simulink library "Damper_Basics"  (R2026a)
settings: Solver=VariableStepAuto
undefined symbols (not defined in the file): Damper, Vehicle
libraries: fl_lib x13, nesl_utility x8, $bdroot x6, sdl_lib x1
Description:
  | Component of Simscape Vehicle Templates Library
  | 
  | Copyright 2018-2026 The MathWorks, Inc.
settings Model: Creator=smiller  LastModifiedBy=smiller

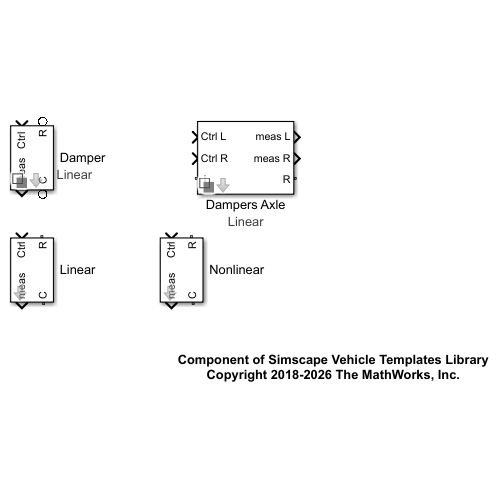
[thumbnail: Simulink's stored preview of the top-level diagram]
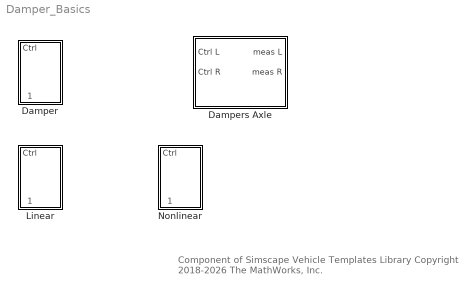
== system Damper_Basics ==
  note: Component of Simscape Vehicle Templates Library
      | Copyright 2018-2026 The MathWorks, Inc.
  Damper : Subsystem  Variant=on  VariantControlMode=label  VariantControl=Variant1  LabelModeActiveChoice=Linear  mask(Variants for Damper){Damper=Vehicle.Chassis.Damper.Axle1, VariantLabel=Vehicle.Chassis.Damper.Axle1.class.Value, InitTriggerDropdown=1}
      mask prompts: Damper "Damper Parameters"; VariantLabel "Variant Label"; InitTriggerDropdown "Initialization Trigger Dropdown"
      mask help: Select option and provide parameters for damper. Option is chosen by string provided in Variant Label. The parameters for the selected option is contained in Damper data structure.
      mask init:
      | curblk = gcb;
      | 
      | % Set variant for this block 
      | set_param(curblk,'LabelModeActiveChoice',VariantLabel);
      | 
      | % Trigger Mask Initialization for 
      | % variant subsystems below this level
      | sm_car_lib_maskInitTrigger(curblk);
      settings: AttributesFormatString=%<ActiveVariant>
      mask TypeOptions InitTriggerDropdown: 0 | 1
      mask Display: disp(' ')
  Dampers Axle : Subsystem  Variant=on  VariantControlMode=label  VariantControl=Variant1  LabelModeActiveChoice=Linear  mask(Variants for Dampers){Damper=Vehicle.Chassis.Damper.Axle1, VariantLabel=Vehicle.Chassis.Damper.Axle1.class.Value, InitTriggerDropdown=1}
      mask prompts: Damper "Damper Parameters"; VariantLabel "Variant Label"; InitTriggerDropdown "Initialization Trigger Dropdown"
      mask help: Select option and provide parameters for left and right dampers. Option is chosen by string provided in Variant Label. The parameters for the selected option is contained in Damper data structure.
      mask init:
      | curblk = gcb;
      | 
      | % Set variant for this block 
      | set_param(curblk,'LabelModeActiveChoice',VariantLabel);
      | 
      | % Trigger Mask Initialization for 
      | % variant subsystems below this level
      | sm_car_lib_maskInitTrigger(curblk);
      settings: AttributesFormatString=%<ActiveVariant>
      mask TypeOptions InitTriggerDropdown: 0 | 1
      mask Display: disp(' ')
  Linear : Subsystem  VariantControl=Linear  mask(Linear Damper with Bumpstop){dam_b=Damper.Damping.d.Value, hp_dpr_top=Damper.Damping.sTop.Value, hp_dpr_bot=Damper.Damping.sBottom.Value, bs_lim_upper=Damper.Endstop.xMax.Value, bs_lim_lower=Damper.Endstop.xMin.Value, bs_k_upper=Damper.Endstop.KxMax.Value, bs_k_lower=Damper.Endstop.KxMin.Value, bs_b_upper=Damper.Endstop.dxMax.Value, bs_b_lower=Damper.Endstop.dxMin.Value, bs_region=Damper.Endstop.xTransition.Value}
      mask prompts: dam_b "Damper (N/(m/s))"; hp_dpr_top "HP Damper Top [xyz] (m)"; hp_dpr_bot "HP Damper Bottom [xyz] (m)"; bs_region "Transition Region (m)"
      mask help: Linear damper with bumpstop at top and bottom.
      mask init:
      | dam_x0 = norm(hp_dpr_top - hp_dpr_bot);
      mask TypeOptions dam_b: Damper/D
      mask DialogControl text_bumpstop_upper Prompt: Upper
      mask DialogControl text_bumpstop_lower Prompt: Lower
      mask DialogControl text_bumpstop_limit Prompt: Limit (m)
      mask DialogControl text_bumpstop_k Prompt: Stiffness (N/m)
      mask DialogControl text_bumpstop_b Prompt: Damping  (N/(m/s))
  Nonlinear : Subsystem  VariantControl=Nonlinear  mask(Nonlinear Damper with Bumpstop){velocity_vector=Damper.Damping.vDamper.Value, force_vector=Damper.Damping.fDamper.Value, hp_dpr_top=Damper.Damping.sTop.Value, hp_dpr_bot=Damper.Damping.sBottom.Value, bs_lim_upper=Damper.Endstop.xMax.Value, bs_lim_lower=Damper.Endstop.xMin.Value, bs_k_upper=Damper.Endstop.KxMax.Value, bs_k_lower=Damper.Endstop.KxMin.Value, bs_b_upper=Damper.Endstop.dxMax.Value, bs_b_lower=Damper.Endstop.dxMin.Value, bs_region=Damper.Endstop.xTransition.Value}
      mask prompts: velocity_vector "Velocity vector"; force_vector "Force vector"; hp_dpr_top "HP Damper Top [xyz] (m)"; hp_dpr_bot "HP Damper Bottom [xyz] (m)"; bs_region "Transition Region (m)"
      mask help: Damper with damping coefficient specified as a lookup table in parallel with a bumpstop.
      mask init:
      | dam_x0 = norm(hp_dpr_top - hp_dpr_bot);
      mask TypeOptions velocity_vector: Damper/velocity_vector
      mask TypeOptions force_vector: Damper/force_vector
      mask DialogControl text_bumpstop_upper Prompt: Upper
      mask DialogControl text_bumpstop_lower Prompt: Lower
      mask DialogControl text_bumpstop_limit Prompt: Limit (m)
      mask DialogControl text_bumpstop_k Prompt: Stiffness (N/m)
      mask DialogControl text_bumpstop_b Prompt: Damping  (N/(m/s))

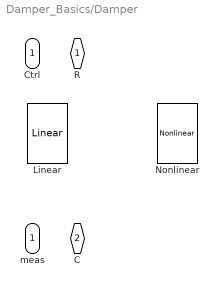
== system Damper_Basics/Damper ==
  "Ctrl " : Inport
  Linear : $bdroot/Linear  VariantControl=Linear  dam_b=Damper.Damping.d.Value  hp_dpr_top=Damper.Damping.sTop.Value  hp_dpr_bot=Damper.Damping.sBottom.Value  bs_lim_upper=Damper.Endstop.xMax.Value  bs_lim_lower=Damper.Endstop.xMin.Value  bs_k_upper=Damper.Endstop.KxMax.Value  bs_k_lower=Damper.Endstop.KxMin.Value  bs_b_upper=Damper.Endstop.dxMax.Value  bs_b_lower=Damper.Endstop.dxMin.Value  bs_region=Damper.Endstop.xTransition.Value
  Nonlinear : $bdroot/Nonlinear  VariantControl=Nonlinear  velocity_vector=Damper.Damping.vDamper.Value  force_vector=Damper.Damping.fDamper.Value  hp_dpr_top=Damper.Damping.sTop.Value  hp_dpr_bot=Damper.Damping.sBottom.Value  bs_lim_upper=Damper.Endstop.xMax.Value  bs_lim_lower=Damper.Endstop.xMin.Value  bs_k_upper=Damper.Endstop.KxMax.Value  bs_k_lower=Damper.Endstop.KxMin.Value  bs_b_upper=Damper.Endstop.dxMax.Value  bs_b_lower=Damper.Endstop.dxMin.Value  bs_region=Damper.Endstop.xTransition.Value
  " R" : PMIOPort  Side=Left
  " C" : PMIOPort  Port=2  Side=Right
  " meas" : Outport  VectorParamsAs1DForOutWhenUnconnected=off

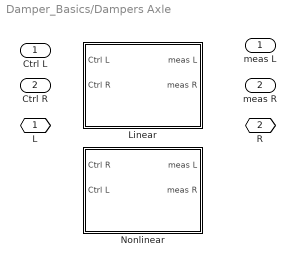
== system Damper_Basics/Dampers Axle ==
  "Ctrl L " : Inport
  "Ctrl R " : Inport  Port=2
  Linear : Subsystem  VariantControl=Linear
  Nonlinear : Subsystem  VariantControl=Nonlinear
  " L" : PMIOPort  Side=Left
  " R" : PMIOPort  Port=2  Side=Right
  " meas L" : Outport  VectorParamsAs1DForOutWhenUnconnected=off
  " meas R" : Outport  Port=2  VectorParamsAs1DForOutWhenUnconnected=off

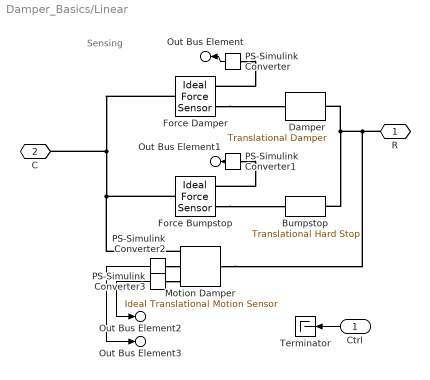
== system Damper_Basics/Linear ==
  note: Sensing
  Ctrl : Inport
  Bumpstop : fl_lib/Mechanical/Translational Elements/Translational Hard Stop  upper_bnd=bs_lim_upper m  lower_bnd=bs_lim_lower m  model=1  stiff_up=bs_k_upper N/m  stiff_low=bs_k_lower N/m  D_up=bs_b_upper N/(m/s)  D_low=bs_b_lower N/(m/s)  transition=bs_region m  coeff_rest=0.7  v_tol=0.001 m/s  f_tol=0.001 N  v_specify=off  v_priority=None  v=0 m/s  v_nominal_specify=off  v_nominal_value=1  v_nominal_unit=m/s  f_specify=off  f_priority=None  f=0 N  f_nominal_specify=off  f_nominal_value=1  f_nominal_unit=N  x_specify=off  x_priority=High  x=0 m  x_nominal_specify=off  x_nominal_value=1  x_nominal_unit=m  M_specify=off  M_priority=None  M=0
  Damper : fl_lib/Mechanical/Translational Elements/Translational Damper  D=dam_b N/(m/s)  v_specify=off  v_priority=None  v=0 m/s  v_nominal_specify=off  v_nominal_value=1  v_nominal_unit=m/s  f_specify=off  f_priority=None  f=0 N  f_nominal_specify=off  f_nominal_value=1  f_nominal_unit=N
  Force Bumpstop : fl_lib/Mechanical/Mechanical Sensors/Ideal Force Sensor
  Force Damper : fl_lib/Mechanical/Mechanical Sensors/Ideal Force Sensor
  Motion Damper : fl_lib/Mechanical/Mechanical Sensors/Ideal Translational Motion Sensor  reference=foundation.enum.MeasurementReference.difference  acceleration_port=false  velocity_port=true  position_port=true  offset=dam_x0 m
  PS-Simulink Converter : nesl_utility/PS-Simulink Converter  PhysicalDomain=network_engine_domain  SubClassName=ps_output  LeftPortType=input  RightPortType=output  PseudoPeriodic=off  Frequencies=[]  VectorFormat=1-D array  Unit=N  AffineConversion=off
  PS-Simulink Converter1 : nesl_utility/PS-Simulink Converter  PhysicalDomain=network_engine_domain  SubClassName=ps_output  LeftPortType=input  RightPortType=output  PseudoPeriodic=off  Frequencies=[]  VectorFormat=1-D array  Unit=N  AffineConversion=off
  PS-Simulink Converter2 : nesl_utility/PS-Simulink Converter  PhysicalDomain=network_engine_domain  SubClassName=ps_output  LeftPortType=input  RightPortType=output  PseudoPeriodic=off  Frequencies=[]  VectorFormat=1-D array  Unit=m/s  AffineConversion=off
  PS-Simulink Converter3 : nesl_utility/PS-Simulink Converter  PhysicalDomain=network_engine_domain  SubClassName=ps_output  LeftPortType=input  RightPortType=output  PseudoPeriodic=off  Frequencies=[]  VectorFormat=1-D array  Unit=m  AffineConversion=off
  Terminator : Terminator
  R : PMIOPort  Side=Left
  C : PMIOPort  Port=2  Side=Right
  Out Bus Element : Outport  VectorParamsAs1DForOutWhenUnconnected=off  PortName=meas  Element=FDamper
  Out Bus Element1 : Outport  VectorParamsAs1DForOutWhenUnconnected=off  PortName=meas  Element=FBumpstop
  Out Bus Element2 : Outport  VectorParamsAs1DForOutWhenUnconnected=off  PortName=meas  Element=xDamper
  Out Bus Element3 : Outport  VectorParamsAs1DForOutWhenUnconnected=off  PortName=meas  Element=vDamper
  wires:
  Ctrl/1 -> Terminator/1
  PS-Simulink Converter/1 -> Out Bus Element/1
  PS-Simulink Converter2/1 -> Out Bus Element3/1
  PS-Simulink Converter3/1 -> Out Bus Element2/1
  PS-Simulink Converter1/1 -> Out Bus Element1/1
  connections:
  Motion Damper/RConn1 -- Force Bumpstop/LConn1 -- C/RConn1 -- Force Damper/LConn1
  PS-Simulink Converter2/LConn1 -- Motion Damper/RConn2
  PS-Simulink Converter1/LConn1 -- Force Bumpstop/RConn2
  PS-Simulink Converter3/LConn1 -- Motion Damper/RConn3
  PS-Simulink Converter/LConn1 -- Force Damper/RConn2
  Force Bumpstop/RConn1 -- Bumpstop/RConn1
  Force Damper/RConn1 -- Damper/RConn1
  Damper/LConn1 -- Bumpstop/LConn1 -- Motion Damper/LConn1 -- R/RConn1

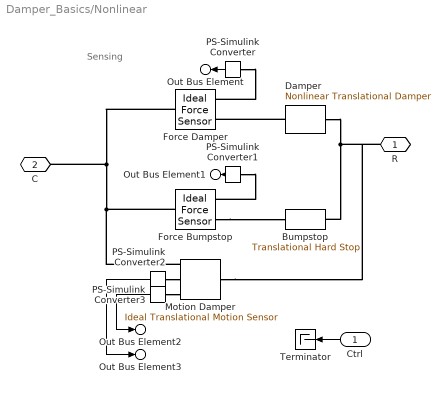
== system Damper_Basics/Nonlinear ==
  note: Sensing
  Ctrl : Inport
  Bumpstop : fl_lib/Mechanical/Translational Elements/Translational Hard Stop  upper_bnd=bs_lim_upper m  lower_bnd=bs_lim_lower m  model=1  stiff_up=bs_k_upper N/m  stiff_low=bs_k_lower N/m  D_up=bs_b_upper N/(m/s)  D_low=bs_b_lower N/(m/s)  transition=bs_region m  coeff_rest=0.7  v_tol=0.001 m/s  f_tol=0.001 N  v_specify=off  v_priority=None  v=0 m/s  v_nominal_specify=off  v_nominal_value=1  v_nominal_unit=m/s  f_specify=off  f_priority=None  f=0 N  f_nominal_specify=off  f_nominal_value=1  f_nominal_unit=N  x_specify=off  x_priority=High  x=0 m  x_nominal_specify=off  x_nominal_value=1  x_nominal_unit=m  M_specify=off  M_priority=None  M=0
  Damper : sdl_lib/Couplings & Drives/Springs & Dampers/Nonlinear Translational Damper  parameterization=2  symmetry=1  coefficient_vector=[10, 0, 1, 0, .1] N/(m/s)  extension_coefficient_vector=[10, 0, 1, 0, .1] N/(m/s)  contraction_coefficient_vector=[100, -1, 10, 0, 0] N/(m/s)  velocity_vector=velocity_vector m/s  force_vector=force_vector N  interp_method=simscape.enum.interpolation.linear  extrap_method=simscape.enum.extrapolation.linear
  Force Bumpstop : fl_lib/Mechanical/Mechanical Sensors/Ideal Force Sensor
  Force Damper : fl_lib/Mechanical/Mechanical Sensors/Ideal Force Sensor
  Motion Damper : fl_lib/Mechanical/Mechanical Sensors/Ideal Translational Motion Sensor  reference=foundation.enum.MeasurementReference.difference  acceleration_port=false  velocity_port=true  position_port=true  offset=dam_x0 m
  PS-Simulink Converter : nesl_utility/PS-Simulink Converter  PhysicalDomain=network_engine_domain  SubClassName=ps_output  LeftPortType=input  RightPortType=output  PseudoPeriodic=off  Frequencies=[]  VectorFormat=1-D array  Unit=N  AffineConversion=off
  PS-Simulink Converter1 : nesl_utility/PS-Simulink Converter  PhysicalDomain=network_engine_domain  SubClassName=ps_output  LeftPortType=input  RightPortType=output  PseudoPeriodic=off  Frequencies=[]  VectorFormat=1-D array  Unit=N  AffineConversion=off
  PS-Simulink Converter2 : nesl_utility/PS-Simulink Converter  PhysicalDomain=network_engine_domain  SubClassName=ps_output  LeftPortType=input  RightPortType=output  PseudoPeriodic=off  Frequencies=[]  VectorFormat=1-D array  Unit=m/s  AffineConversion=off
  PS-Simulink Converter3 : nesl_utility/PS-Simulink Converter  PhysicalDomain=network_engine_domain  SubClassName=ps_output  LeftPortType=input  RightPortType=output  PseudoPeriodic=off  Frequencies=[]  VectorFormat=1-D array  Unit=m  AffineConversion=off
  Terminator : Terminator
  R : PMIOPort  Side=Left
  C : PMIOPort  Port=2  Side=Right
  Out Bus Element : Outport  VectorParamsAs1DForOutWhenUnconnected=off  PortName=meas  Element=FDamper
  Out Bus Element1 : Outport  VectorParamsAs1DForOutWhenUnconnected=off  PortName=meas  Element=FBumpstop
  Out Bus Element2 : Outport  VectorParamsAs1DForOutWhenUnconnected=off  PortName=meas  Element=xDamper
  Out Bus Element3 : Outport  VectorParamsAs1DForOutWhenUnconnected=off  PortName=meas  Element=vDamper
  wires:
  PS-Simulink Converter1/1 -> Out Bus Element1/1
  PS-Simulink Converter3/1 -> Out Bus Element2/1
  PS-Simulink Converter2/1 -> Out Bus Element3/1
  PS-Simulink Converter/1 -> Out Bus Element/1
  Ctrl/1 -> Terminator/1
  connections:
  Damper/LConn1 -- R/RConn1 -- Motion Damper/LConn1 -- Bumpstop/LConn1
  Damper/RConn1 -- Force Damper/RConn1
  Force Bumpstop/RConn1 -- Bumpstop/RConn1
  PS-Simulink Converter/LConn1 -- Force Damper/RConn2
  PS-Simulink Converter3/LConn1 -- Motion Damper/RConn3
  PS-Simulink Converter1/LConn1 -- Force Bumpstop/RConn2
  PS-Simulink Converter2/LConn1 -- Motion Damper/RConn2
  Force Damper/LConn1 -- C/RConn1 -- Force Bumpstop/LConn1 -- Motion Damper/RConn1

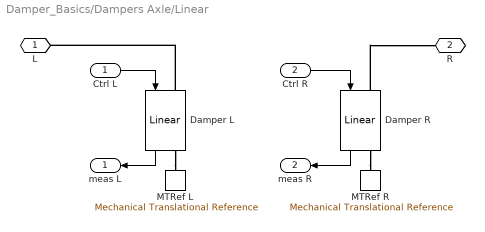
== system Damper_Basics/Dampers Axle/Linear ==
  Ctrl L : Inport
  Ctrl R : Inport  Port=2
  Damper L : $bdroot/Linear  VariantControl=Linear  dam_b=Damper.Damping.d.Value  hp_dpr_top=Damper.Damping.sTop.Value  hp_dpr_bot=Damper.Damping.sBottom.Value  bs_lim_upper=Damper.Endstop.xMax.Value  bs_lim_lower=Damper.Endstop.xMin.Value  bs_k_upper=Damper.Endstop.KxMax.Value  bs_k_lower=Damper.Endstop.KxMin.Value  bs_b_upper=Damper.Endstop.dxMax.Value  bs_b_lower=Damper.Endstop.dxMin.Value  bs_region=Damper.Endstop.xTransition.Value
  Damper R : $bdroot/Linear  VariantControl=Linear  dam_b=Damper.Damping.d.Value  hp_dpr_top=Damper.Damping.sTop.Value  hp_dpr_bot=Damper.Damping.sBottom.Value  bs_lim_upper=Damper.Endstop.xMax.Value  bs_lim_lower=Damper.Endstop.xMin.Value  bs_k_upper=Damper.Endstop.KxMax.Value  bs_k_lower=Damper.Endstop.KxMin.Value  bs_b_upper=Damper.Endstop.dxMax.Value  bs_b_lower=Damper.Endstop.dxMin.Value  bs_region=Damper.Endstop.xTransition.Value
  MTRef L : fl_lib/Mechanical/Translational Elements/Mechanical Translational Reference
  MTRef R : fl_lib/Mechanical/Translational Elements/Mechanical Translational Reference
  " L" : PMIOPort  Side=Left
  " R" : PMIOPort  Port=2  Side=Right
  meas L : Outport  VectorParamsAs1DForOutWhenUnconnected=off
  meas R : Outport  Port=2  VectorParamsAs1DForOutWhenUnconnected=off
  wires:
  Damper L/1 -> meas L/1
  Ctrl L/1 -> Damper L/1
  Ctrl R/1 -> Damper R/1
  Damper R/1 -> meas R/1
  connections:
  Damper L/RConn1 -- MTRef L/LConn1
  Damper R/LConn1 -- " R"/RConn1
  Damper R/RConn1 -- MTRef R/LConn1
  Damper L/LConn1 -- " L"/RConn1

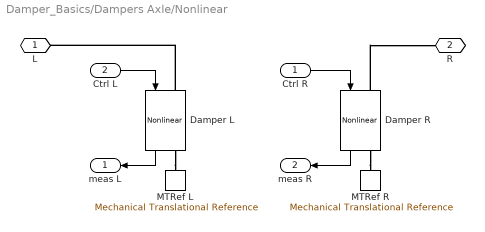
== system Damper_Basics/Dampers Axle/Nonlinear ==
  Ctrl R : Inport
  Ctrl L : Inport  Port=2
  Damper L : $bdroot/Nonlinear  VariantControl=Nonlinear  velocity_vector=Damper.Damping.vDamper.Value  force_vector=Damper.Damping.fDamper.Value  hp_dpr_top=Damper.Damping.sTop.Value  hp_dpr_bot=Damper.Damping.sBottom.Value  bs_lim_upper=Damper.Endstop.xMax.Value  bs_lim_lower=Damper.Endstop.xMin.Value  bs_k_upper=Damper.Endstop.KxMax.Value  bs_k_lower=Damper.Endstop.KxMin.Value  bs_b_upper=Damper.Endstop.dxMax.Value  bs_b_lower=Damper.Endstop.dxMin.Value  bs_region=Damper.Endstop.xTransition.Value
  Damper R : $bdroot/Nonlinear  VariantControl=Nonlinear  velocity_vector=Damper.Damping.vDamper.Value  force_vector=Damper.Damping.fDamper.Value  hp_dpr_top=Damper.Damping.sTop.Value  hp_dpr_bot=Damper.Damping.sBottom.Value  bs_lim_upper=Damper.Endstop.xMax.Value  bs_lim_lower=Damper.Endstop.xMin.Value  bs_k_upper=Damper.Endstop.KxMax.Value  bs_k_lower=Damper.Endstop.KxMin.Value  bs_b_upper=Damper.Endstop.dxMax.Value  bs_b_lower=Damper.Endstop.dxMin.Value  bs_region=Damper.Endstop.xTransition.Value
  MTRef L : fl_lib/Mechanical/Translational Elements/Mechanical Translational Reference
  MTRef R : fl_lib/Mechanical/Translational Elements/Mechanical Translational Reference
  " L" : PMIOPort  Side=Left
  " R" : PMIOPort  Port=2  Side=Right
  meas L : Outport  VectorParamsAs1DForOutWhenUnconnected=off
  meas R : Outport  Port=2  VectorParamsAs1DForOutWhenUnconnected=off
  wires:
  Damper R/1 -> meas R/1
  Ctrl R/1 -> Damper R/1
  Ctrl L/1 -> Damper L/1
  Damper L/1 -> meas L/1
  connections:
  Damper L/LConn1 -- " L"/RConn1
  Damper R/RConn1 -- MTRef R/LConn1
  Damper R/LConn1 -- " R"/RConn1
  Damper L/RConn1 -- MTRef L/LConn1
